simulink model "EventCameraSensor"  (R2020b)
settings: configuration reference "Camera" (kept outside this file)
undefined symbols (not defined in the file): DiscIntNeverNeededParam, imageHeight, imageWidth, ts_camera
libraries: simulink x2, visiongeotforms x1
settings Model: DataDictionary=Dictionary.sldd  EnableAccessToBaseWorkspace=off  Creator=alons  LastModifiedBy=alons
settings ConfigSetRef: SourceName=Camera

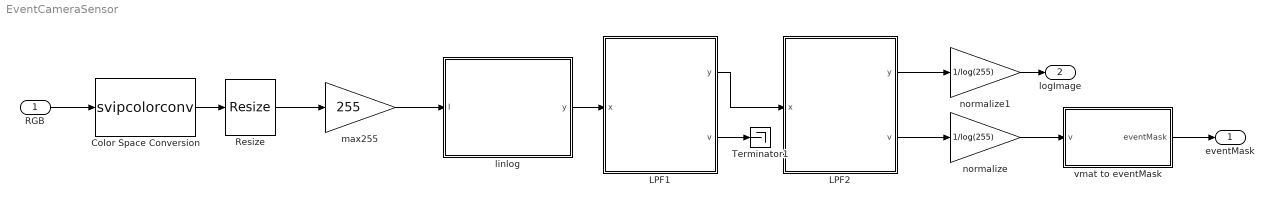
== system EventCameraSensor ==
  RGB : Inport  PortDimensions=[imageHeight,imageWidth,3]
  Color Space Conversion : S-Function  FunctionName=svipcolorconv  Parameters=conversionActive, wp, rec, sys, imagePorts, conversion  SFunctionDeploymentMode=off  EnableBusSupport=off  mask(Color Space Conversion){conversion=Obsolete, conversionActive=R'G'B' to intensity, wp_str=D65, rec=Rec. 601 (SDTV), sys=1125/60/2:1, imagePorts=One multidimensional signal}
      mask prompts: conversion "vision:masks:Conversionobsoleted"; conversionActive "vision:masks:Conversion"; wp_str "vision:masks:WhitePoint"; rec "vision:masks:UseConversionSpecifiedBy"; sys "vision:masks:ScanningStandard"; imagePorts "vision:masks:ImageSignal"
      mask help: vision:masks:ColorSpaceDescription
      mask init:
      | [si, so, blkname] = vipblkcolorconv('icon');
      | wp = whitepoint(get_param(gcbh,'wp_str'));
      mask Help: eval('visionblockhelp');
      mask TypeOptions conversion: R'G'B' to Y'CbCr | Y'CbCr to R'G'B' | R'G'B' to intensity | R'G'B' to HSV | HSV to R'G'B' | sR'G'B' to XYZ | XYZ to sR'G'B' | sR'G'B' to L*a*b* | L*a*b* to sR'G'B' | Obsolete
      mask Callback conversion: vipblkcolorconv;
      mask TypeOptions conversionActive: R'G'B' to Y'CbCr | Y'CbCr to R'G'B' | R'G'B' to intensity | R'G'B' to HSV | HSV to R'G'B' | sR'G'B' to XYZ | XYZ to sR'G'B' | sR'G'B' to L*a*b* | L*a*b* to sR'G'B'
      mask Callback conversionActive: vipblkcolorconv;
      mask TypeOptions wp_str: D50 | D55 | D65
      mask TypeOptions rec: Rec. 601 (SDTV) | Rec. 709 (HDTV)
      mask Callback rec: vipblkcolorconv;
      mask TypeOptions sys: 1125/60/2:1 | 1250/50/2:1
      mask TypeOptions imagePorts: vision:masks:OneMultidimensionalSignal | vision:masks:SeparateColorSignals
      mask Display:
      | disp(blkname)
      | 
      | port_label('input', si(1).port, si(1).txt);
      | port_label('input', si(2).port, si(2).txt);
      | port_label('input', si(3).port, si(3).txt);
      | 
      | 
      | port_label('output',so(1).port, so(1).txt);
      | port_label('output',so(2).port, so(2).txt);
      | port_label('output',so(3).port, so(3).txt);
  LPF1 : Subsystem  mask{PosBW=10}
      mask prompts: PosBW "Position BW [Hz]"
      mask Display: fprintf('Linear LPF %.3g[Hz]',PosBW);
  LPF2 : Subsystem  mask{PosBW=10}
      mask prompts: PosBW "Position BW [Hz]"
      mask Display: fprintf('Linear LPF %.3g[Hz]',PosBW);
  Resize : visiongeotforms/Resize  specify=Output size as a percentage of input size  rfactor=[20 20]  outCols=25  outRows=25  outRowsCols=[25 35]  interp_method=Bilinear  antialias=on  useROI=off  roiFlag=off  roundingMode=Nearest  overflowMode=on  prodOutputMode=Binary point scaling  prodOutputWordLength=32  prodOutputFracLength=10
      settings: SourceProductBaseCode=VP
  Terminator1 : Terminator
  linlog : MATLAB Function  TreatAsAtomicUnit=on  mask{threshold=20}
  max255 : Gain  Gain=255
  normalize : Gain  Gain=1/log(255)
  normalize1 : Gain  Gain=1/log(255)
  vmat to eventMask : Subsystem  mask{threshold=0.01/ts_camera}
  eventMask : Outport
  logImage : Outport  Port=2
  wires:
  LPF2/1(y) -> normalize1/1
  LPF2/2(v) -> normalize/1
  vmat to eventMask/1(eventMask) -> eventMask/1
  normalize/1 -> vmat to eventMask/1(v)
  LPF1/1(y) -> LPF2/1(x)
  LPF1/2(v) -> Terminator1/1
  normalize1/1 -> logImage/1
  Resize/1 -> max255/1
  Color Space Conversion/1 -> Resize/1
  RGB/1 -> Color Space Conversion/1
  linlog/1(y) -> LPF1/1(x)
  max255/1 -> linlog/1(I)

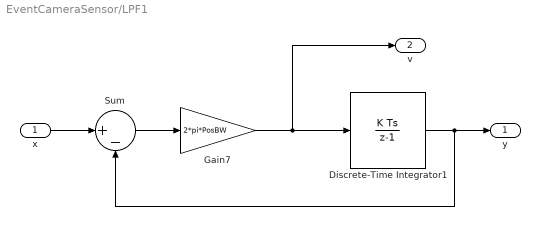
== system EventCameraSensor/LPF1 ==
  x : Inport
  Discrete-Time Integrator1 : DiscreteIntegrator  SampleTime=-1  ICPrevOutput=DiscIntNeverNeededParam  ICPrevScaledInput=DiscIntNeverNeededParam
  Gain7 : Gain  Gain=2*pi*PosBW
  Sum : Sum  Inputs=|+-
  y : Outport  VectorParamsAs1DForOutWhenUnconnected=off
  v : Outport  Port=2  VectorParamsAs1DForOutWhenUnconnected=off
  wires:
  x/1 -> Sum/1
  Sum/1 -> Gain7/1
  Discrete-Time Integrator1/1 -> y/1, Sum/2
  Gain7/1 -> Discrete-Time Integrator1/1, v/1

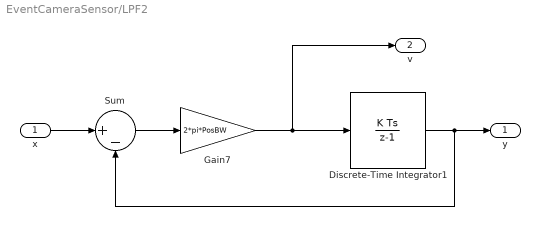
== system EventCameraSensor/LPF2 ==
  x : Inport
  Discrete-Time Integrator1 : DiscreteIntegrator  SampleTime=-1  ICPrevOutput=DiscIntNeverNeededParam  ICPrevScaledInput=DiscIntNeverNeededParam
  Gain7 : Gain  Gain=2*pi*PosBW
  Sum : Sum  Inputs=|+-
  y : Outport  VectorParamsAs1DForOutWhenUnconnected=off
  v : Outport  Port=2  VectorParamsAs1DForOutWhenUnconnected=off
  wires:
  Gain7/1 -> v/1, Discrete-Time Integrator1/1
  Discrete-Time Integrator1/1 -> Sum/2, y/1
  Sum/1 -> Gain7/1
  x/1 -> Sum/1

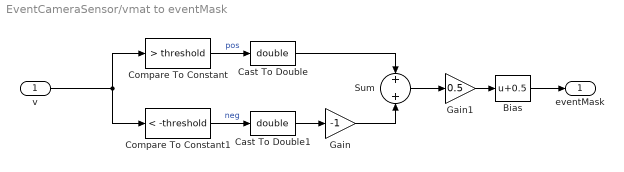
== system EventCameraSensor/vmat to eventMask ==
  v : Inport
  Bias : Bias  Bias=0.5
  Cast To Double : DataTypeConversion  OutDataTypeStr=double
  Cast To Double1 : DataTypeConversion  OutDataTypeStr=double
  Compare To Constant : simulink/Logic and Bit Operations/Compare To Constant  relop=>  const=threshold  OutDataTypeStr=uint8  ZeroCross=off
  Compare To Constant1 : simulink/Logic and Bit Operations/Compare To Constant  relop=<  const=-threshold  OutDataTypeStr=uint8  ZeroCross=off
  Gain : Gain  Gain=-1
  Gain1 : Gain  Gain=0.5
  Sum : Sum  Inputs=+|+
  eventMask : Outport
  wires:
  Gain/1 -> Sum/2
  v/1 -> Compare To Constant/1, Compare To Constant1/1
  Compare To Constant1/1 -> Cast To Double1/1  "neg"
  Cast To Double1/1 -> Gain/1
  Compare To Constant/1 -> Cast To Double/1  "pos"
  Cast To Double/1 -> Sum/1
  Sum/1 -> Gain1/1
  Gain1/1 -> Bias/1
  Bias/1 -> eventMask/1

== matlab function EventCameraSensor/linlog ==
  data: I input double; y output; threshold parameter double
function y = linlogfn(I,threshold) %codegen
%returns value in range of 0-log(255) -> 0-5.55413
%taken from "Event-Based Angular Velocity Regression with Spiking Networks"
f = (1/threshold)*log(threshold);
mask = I>threshold;
y=zeros(size(I));
for ii=1:numel(I)
   if mask(ii)
       y(ii) = log(I(ii));
   else
       y(ii) = I(ii)*f;
   end
end
end
